simulink model "SoCesti"  (R2025a)
settings: Solver=FixedStepAuto  StartTime=0.0  StopTime=37660  FixedStep=1  RelTol=1e-3
values from neighbouring files (symbols this model uses):
  dOCV_dSOC_25 = [27.0351343549 21.2513205156 13.5820163963 10.6101110655 8.83642238875 7.64097964374 6.7848233075 6.15584045027 5.63144355991 5.17465177199 4.80430871102 4.47325692957 ... (201 elements, 1x201)]    [WSN9.mat]
  OCV_25 = [3.02032761574 3.15550328751 3.23284082089 3.29132345148 3.33894193155 3.37968767536 3.41535172799 3.44753590844 3.47691013249 3.50385034404 3.52865665021 3.55189343115 ... (201 elements, 1x201)]    [WSN9.mat]
  SOC = [0 0.005 0.01 0.015 0.02 0.025 0.03 0.035 0.04 0.045 0.05 0.055 ... (201 elements, 1x201)]    [WSN9.mat]
libraries: matrix_library x6
settings Model: Creator=lty32  LastModifiedBy=lty32
settings OptimizationCC: DefaultParameterBehavior=Inlined  EnhancedBackFolding=on  PassReuseOutputArgsThreshold=0.0  OptimizeBlockOrder=speed  DifferentSizesBufferReuse=on  OptimizationCustomize=off
settings DebuggingCC: ParameterTunabilityLossMsg=error  SFUnexpectedBacktrackingDiag=warning  SFNoUnconditionalDefaultTransitionDiag=warning
settings SFSimCC: MATLABDynamicMemAlloc=off
settings RTWCC: GenerateReport=on  BuildConfiguration=Debug  LaunchReport=on
settings CodeAppCC: ForceParamTrailComments=on  OperatorAnnotations=on  EnableCustomComments=on

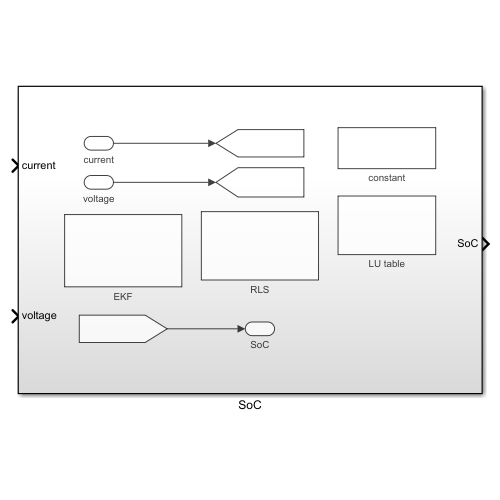
[thumbnail: Simulink's stored preview of the top-level diagram]
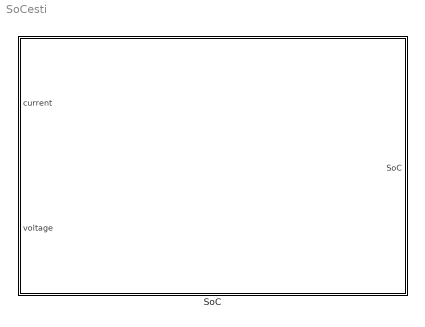
== system SoCesti ==
  SoC : Subsystem

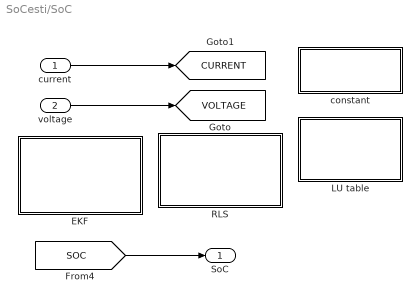
== system SoCesti/SoC ==
  current : Inport
  voltage : Inport  Port=2
  EKF : Subsystem
  LU table : Subsystem
  RLS : Subsystem
  constant : Subsystem
  SoC : Outport
  tag scope: CURRENT=global, VOLTAGE=global
  wires:
  current/1 -> [CURRENT]
  voltage/1 -> [VOLTAGE]
  [SOC] -> SoC/1

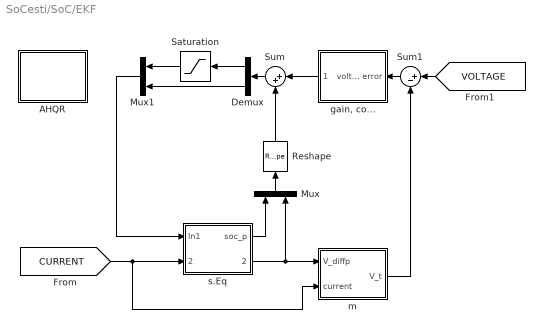
== system SoCesti/SoC/EKF ==
  AHQR : Subsystem
  Demux : Demux  Outputs=2
  Mux : Mux  Inputs=2
  Mux1 : Mux  Inputs=2
  Reshape : Reshape  OutputDimensionality=Column vector (2-D)
  Saturation : Saturate  UpperLimit=1  LowerLimit=0
  Sum : Sum  Inputs=|++
  Sum1 : Sum  Inputs=|+-
  "gain, co..." : Subsystem
  m : Subsystem
  s.Eq : Subsystem
  wires:
  [CURRENT] -> m/2(current), s.Eq/2(current)
  s.Eq/2(V_diffp) -> m/1(V_diffp), Mux/2
  Mux/1 -> Reshape/1
  Reshape/1 -> Sum/2
  Saturation/1 -> Mux1/1
  Demux/1 -> Saturation/1
  Demux/2 -> Mux1/2
  Sum/1 -> Demux/1
  Mux1/1 -> s.Eq/1(In1)
  "gain, co..."/1(1) -> Sum/1
  Sum1/1 -> "gain, co..."/1(voltage error)
  [VOLTAGE] -> Sum1/1
  s.Eq/1(soc_p) -> Mux/1
  m/1(V_t) -> Sum1/2

== system SoCesti/SoC/LU table ==
  1-D Lookup Table1 : Lookup_n-D  NumberOfTableDimensions=1  BreakpointsForDimension1=SOC  Table=OCV_25  InternalRulePriority=Speed  RndMeth=Simplest
  1-D Lookup Table4 : Lookup_n-D  NumberOfTableDimensions=1  BreakpointsForDimension1=SOC  Table=dOCV_dSOC_25  InternalRulePriority=Speed  RndMeth=Simplest
  tag scope: OCV=global, dOCV=global
  wires:
  [SOC] -> 1-D Lookup Table4/1, 1-D Lookup Table1/1
  1-D Lookup Table1/1 -> [OCV]
  1-D Lookup Table4/1 -> [dOCV]

== system SoCesti/SoC/RLS ==
  Subsystem : Subsystem
  tag scope: C1=global, R0=global, R1=global
  wires:
  Subsystem/1(r0) -> [R0]
  Subsystem/2(r1) -> [R1]
  Subsystem/3(c1) -> [C1]
  [VOLTAGE] -> Subsystem/2(voltage)
  [CURRENT] -> Subsystem/1(current)

== system SoCesti/SoC/constant ==
  "[C]" : Constant  Value=5.1344*3600  VectorParams1D=off
  sampling time [s] : Constant  VectorParams1D=off
  tag scope: dt=global, q=global
  wires:
  sampling time [s]/1 -> [dt]
  "[C]"/1 -> [q]

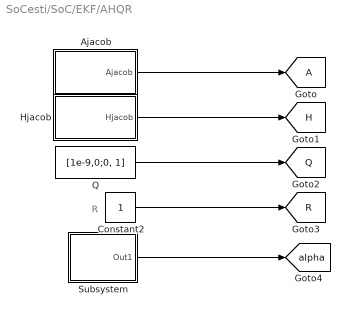
== system SoCesti/SoC/EKF/AHQR ==
  note: R
  Ajacob : Subsystem
  Constant2 : Constant  VectorParams1D=off
  Goto : Goto  TagVisibility=global
  Hjacob : Subsystem
  Q : Constant  Value=[1e-9,0;0, 1]  VectorParams1D=off
  Subsystem : Subsystem
  tag scope: H=global, Q=global, R=global, alpha=global
  wires:
  Hjacob/1(Hjacob) -> [H]
  Ajacob/1(Ajacob) -> Goto/1
  Q/1 -> [Q]
  Constant2/1 -> [R]
  Subsystem/1(Out1) -> [alpha]

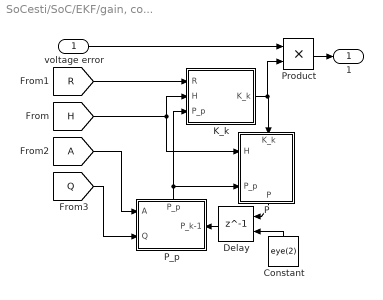
== system SoCesti/SoC/EKF/gain, co... ==
  voltage error : Inport
  Constant : Constant  Value=eye(2)  VectorParams1D=off
  Delay : Delay  DelayLength=1  InitialConditionSource=Input port  InitialCondition=0
      settings: InputPortMap=u0,p4
  From2 : From  TagVisibility=global
  K_k : Subsystem
  P : Subsystem
      settings: PortSchema="{\"entries\":[{\"content\":{\"sides\":[{\"content\":{\"connectorIds\":[\"In1\"]},\"type\":\"ConnectorPlacement.EquallySpacedRectSide\",\"uuid\":\"6f300193-b535-4daf-8653-539d9fbd6dc4\"},{\"content\":{\"connectorIds\":[\"Out1\"],\"side\":\"RIGHT\"},\"type\":\"ConnectorPlacement.EquallySpacedRectSide\",\"uuid\":\"87a1046a-ef69-4257-b5a0-a19886caf6fd\"},{\"content\":{\"connectorIds\":[\"In2\",\"In3\"],\"side\":\"TOP\"},\"type\":\"ConnectorPlacement.EquallySpacedRectSide\",\"uuid\":\"b6a053fa-a3d4-4df4-83df-54ae82e90296\"},{\"content\":{\"side\":\"BOTTOM\"},\"type\":\"ConnectorPlacement.EquallySpacedRectSide\",\"uuid\":\"c9b75463-d757-4499-9316-63b6258cebf3\"}]},\"type\":\"ConnectorPlacement.EquallySpacedConnector\",\"uuid\":\"417e791e-5d64-4019-ac72-5f0d428a58a7\"}],\"packageUris\":[\"http://schema.mathworks.com/mf0/Connector/R2020b\"],\"version\":\"1.0\"}"
  P_p : Subsystem
      settings: PortSchema="{\"entries\":[{\"content\":{\"sides\":[{\"content\":{\"connectorIds\":[\"In1\"]},\"type\":\"ConnectorPlacement.EquallySpacedRectSide\",\"uuid\":\"6f300193-b535-4daf-8653-539d9fbd6dc4\"},{\"content\":{\"connectorIds\":[\"In2\",\"In3\"],\"side\":\"RIGHT\"},\"type\":\"ConnectorPlacement.EquallySpacedRectSide\",\"uuid\":\"87a1046a-ef69-4257-b5a0-a19886caf6fd\"},{\"content\":{\"connectorIds\":[\"Out1\"],\"side\":\"TOP\"},\"type\":\"ConnectorPlacement.EquallySpacedRectSide\",\"uuid\":\"b6a053fa-a3d4-4df4-83df-54ae82e90296\"}]},\"type\":\"ConnectorPlacement.EquallySpacedConnector\",\"uuid\":\"417e791e-5d64-4019-ac72-5f0d428a58a7\"}],\"packageUris\":[\"http://schema.mathworks.com/mf0/Connector/R2020b\"],\"version\":\"1.0\"}"
  Product : Product
  1 : Outport
  wires:
  P/1(P) -> Delay/1
  K_k/1(K_k) -> P/1(K_k), Product/2
  P_p/1(P_p) -> K_k/3(P_p), P/3(P_p)
  [R] -> K_k/1(R)
  [H] -> K_k/2(H), P/2(H)
  [Q] -> P_p/3(Q)
  voltage error/1 -> Product/1
  From2/1 -> P_p/2(A)
  Delay/1 -> P_p/1(P_k-1)
  Constant/1 -> Delay/2
  Product/1 -> 1/1

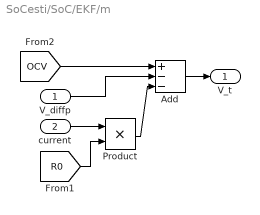
== system SoCesti/SoC/EKF/m ==
  V_diffp : Inport
  current : Inport  Port=2
  Add : Sum  Inputs=+--
  Product : Product
  V_t : Outport
  wires:
  Add/1 -> V_t/1
  [OCV] -> Add/1
  V_diffp/1 -> Add/2
  [R0] -> Product/2
  current/1 -> Product/1
  Product/1 -> Add/3

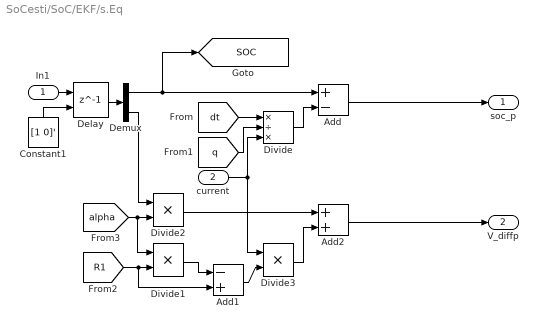
== system SoCesti/SoC/EKF/s.Eq ==
  In1 : Inport
  current : Inport  Port=2
  Add : Sum  Inputs=+-
  Add1 : Sum  Inputs=-+
  Add2 : Sum
  Constant1 : Constant  Value=[1 0]'  VectorParams1D=off
  Delay : Delay  DelayLength=1  InitialConditionSource=Input port  InitialCondition=0
      settings: InputPortMap=u0,p4
  Demux : Demux  Outputs=2
  Divide : Product  Inputs=*/*
  Divide1 : Product  Inputs=**
  Divide2 : Product  Inputs=**
  Divide3 : Product  Inputs=**
  soc_p : Outport
  V_diffp : Outport  Port=2
  tag scope: SOC=global
  wires:
  current/1 -> Divide3/1, Divide/3
  [dt] -> Divide/1
  [q] -> Divide/2
  Divide/1 -> Add/2
  Demux/1 -> [SOC], Add/1
  Add/1 -> soc_p/1
  Add2/1 -> V_diffp/1
  In1/1 -> Delay/1
  Delay/1 -> Demux/1
  Constant1/1 -> Delay/2
  [R1] -> Add1/2, Divide1/2
  [alpha] -> Divide1/1, Divide2/2
  Demux/2 -> Divide2/1
  Divide1/1 -> Add1/1
  Divide2/1 -> Add2/1
  Add1/1 -> Divide3/2
  Divide3/1 -> Add2/2

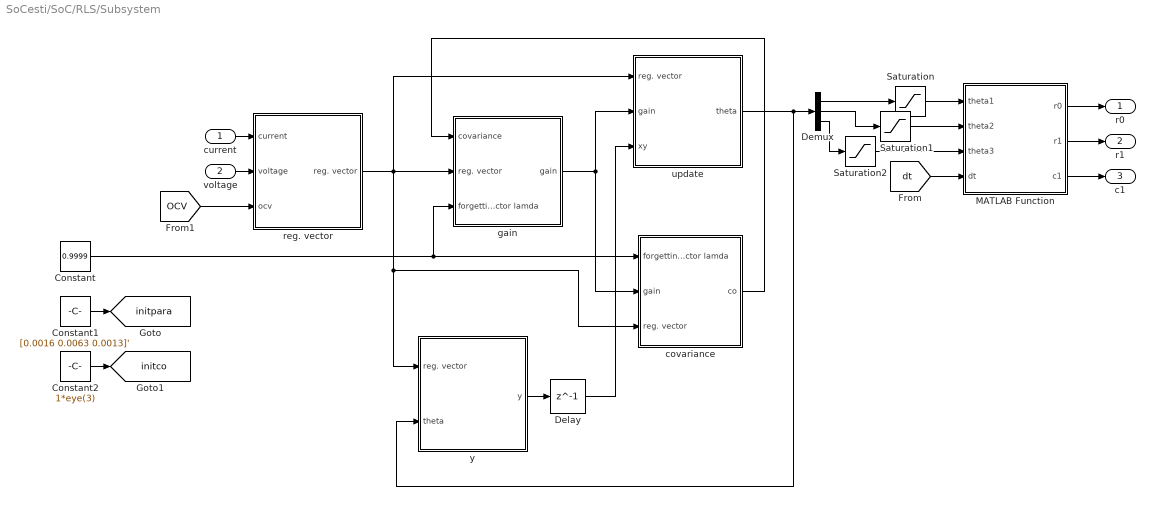
== system SoCesti/SoC/RLS/Subsystem ==
  current : Inport
  voltage : Inport  Port=2
  Constant : Constant  Value=0.9999
  Constant1 : Constant  Value=[0.0016 0.0063 0.0013]'  VectorParams1D=off
  Constant2 : Constant  Value=1*eye(3)  VectorParams1D=off
  Delay : Delay  DelayLength=1  InitialCondition=0
  Demux : Demux  Outputs=3
  MATLAB Function : MATLAB Function  TreatAsAtomicUnit=on
  Saturation : Saturate  UpperLimit=0.1  LowerLimit=0.000001  LinearizeAsGain=off
  Saturation1 : Saturate  LowerLimit=0.000001
  Saturation2 : Saturate  LowerLimit=0.000001
  covariance : Subsystem
  gain : Subsystem
  reg. vector : Subsystem
  update : Subsystem
  y : Subsystem
  r0 : Outport
  r1 : Outport  Port=2
  c1 : Outport  Port=3
  tag scope: initco=global, initpara=global
  wires:
  current/1 -> reg. vector/1(current)
  voltage/1 -> reg. vector/2(voltage)
  MATLAB Function/1(r0) -> r0/1
  MATLAB Function/2(r1) -> r1/1
  MATLAB Function/3(c1) -> c1/1
  [dt] -> MATLAB Function/4(dt)
  update/1(theta) -> y/2(theta), Demux/1
  reg. vector/1(reg. vector) -> y/1(reg. vector), covariance/3(reg. vector), update/1(reg. vector), gain/2(reg. vector)
  covariance/1(co) -> gain/1(covariance)
  gain/1(gain) -> covariance/2(gain), update/2(gain)
  Constant/1 -> gain/3(forgetting factor lamda), covariance/1(forgetting factor lamda)
  Constant1/1 -> [initpara]
  Constant2/1 -> [initco]
  [OCV] -> reg. vector/3(ocv)
  Demux/1 -> Saturation/1
  Saturation/1 -> MATLAB Function/1(theta1)
  Saturation1/1 -> MATLAB Function/2(theta2)
  Demux/2 -> Saturation1/1
  Saturation2/1 -> MATLAB Function/3(theta3)
  Demux/3 -> Saturation2/1
  y/1(y) -> Delay/1
  Delay/1 -> update/3(xy)

== system SoCesti/SoC/EKF/AHQR/Ajacob ==
  Add : Sum
  Constant : Constant  Value=[0, 0; 0, 1]
  Constant1 : Constant  Value=[1, 0; 0, 0]
  Product : Product
  Ajacob : Outport
  wires:
  Add/1 -> Ajacob/1
  Product/1 -> Add/1
  Constant1/1 -> Add/2
  [alpha] -> Product/2
  Constant/1 -> Product/1

== system SoCesti/SoC/EKF/AHQR/Hjacob ==
  Add : Sum  Inputs=+-
  Constant : Constant  Value=[1 0]  VectorParams1D=off
  Constant1 : Constant  Value=[0 1]  VectorParams1D=off
  Product : Product
  Hjacob : Outport
  wires:
  Add/1 -> Hjacob/1
  Product/1 -> Add/1
  Constant1/1 -> Add/2
  [dOCV] -> Product/2
  Constant/1 -> Product/1

== system SoCesti/SoC/EKF/AHQR/Subsystem ==
  Constant : Constant  Value=-1  VectorParams1D=off
  Divide : Product  Inputs=**//
  Math Function : Math  OutputSignalType=real
  Out1 : Outport
  wires:
  [C1] -> Divide/4
  [R1] -> Divide/3
  [dt] -> Divide/2
  Constant/1 -> Divide/1
  Divide/1 -> Math Function/1
  Math Function/1 -> Out1/1

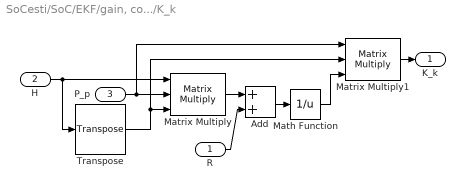
== system SoCesti/SoC/EKF/gain, co.../K_k ==
  R : Inport
  H : Inport  Port=2
  P_p : Inport  Port=3
  Add : Sum
  Math Function : Math  Operator=reciprocal
  Matrix Multiply : Product  Inputs=3  Multiplication=Matrix(*)
  Matrix Multiply1 : Product  Inputs=3  Multiplication=Matrix(*)
  Transpose : matrix_library/Transpose
  K_k : Outport
  wires:
  P_p/1 -> Matrix Multiply1/1, Matrix Multiply/2
  H/1 -> Transpose/1, Matrix Multiply/1
  Transpose/1 -> Matrix Multiply/3, Matrix Multiply1/2
  Matrix Multiply/1 -> Add/1
  R/1 -> Add/2
  Matrix Multiply1/1 -> K_k/1
  Add/1 -> Math Function/1
  Math Function/1 -> Matrix Multiply1/3

== system SoCesti/SoC/EKF/gain, co.../P ==
  K_k : Inport
  H : Inport  Port=2
  P_p : Inport  Port=3
  Matrix Multiply : Product  Inputs=3  Multiplication=Matrix(*)
  Subtract : Sum  Inputs=+-
  P : Outport
  wires:
  K_k/1 -> Matrix Multiply/1
  H/1 -> Matrix Multiply/2
  P_p/1 -> Subtract/1, Matrix Multiply/3
  Matrix Multiply/1 -> Subtract/2
  Subtract/1 -> P/1

== system SoCesti/SoC/EKF/gain, co.../P_p ==
  P_k-1 : Inport
  A : Inport  Port=2
  Q : Inport  Port=3
  Add : Sum
  Matrix Multiply : Product  Inputs=3  Multiplication=Matrix(*)
  Transpose : matrix_library/Transpose
  P_p : Outport
  wires:
  P_k-1/1 -> Matrix Multiply/2
  Q/1 -> Add/2
  A/1 -> Transpose/1, Matrix Multiply/1
  Matrix Multiply/1 -> Add/1
  Transpose/1 -> Matrix Multiply/3
  Add/1 -> P_p/1

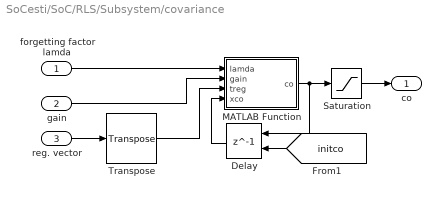
== system SoCesti/SoC/RLS/Subsystem/covariance ==
  forgetting factor lamda : Inport
  gain : Inport  Port=2
  reg. vector : Inport  Port=3
  Delay : Delay  DelayLength=1  InitialConditionSource=Input port  InitialCondition=0
      settings: InputPortMap=u0,p4
  MATLAB Function : MATLAB Function  TreatAsAtomicUnit=on
  Saturation : Saturate  UpperLimit=inf  LowerLimit=0.000001  LinearizeAsGain=off
  Transpose : matrix_library/Transpose
  co : Outport
  wires:
  forgetting factor lamda/1 -> MATLAB Function/1(lamda)
  gain/1 -> MATLAB Function/2(gain)
  reg. vector/1 -> Transpose/1
  Transpose/1 -> MATLAB Function/3(treg)
  MATLAB Function/1(co) -> Saturation/1, Delay/1
  Delay/1 -> MATLAB Function/4(xco)
  [initco] -> Delay/2
  Saturation/1 -> co/1

== system SoCesti/SoC/RLS/Subsystem/gain ==
  covariance : Inport
  reg. vector : Inport  Port=2
  forgetting factor lamda : Inport  Port=3
  Delay : Delay  DelayLength=1  InitialCondition=0
  MATLAB Function : MATLAB Function  TreatAsAtomicUnit=on
  Transpose : matrix_library/Transpose
  gain : Outport
  wires:
  forgetting factor lamda/1 -> MATLAB Function/1(lamda)
  reg. vector/1 -> MATLAB Function/2(reg), Transpose/1
  Transpose/1 -> MATLAB Function/3(treg)
  covariance/1 -> Delay/1
  Delay/1 -> MATLAB Function/4(xco)
  MATLAB Function/1(gain) -> gain/1

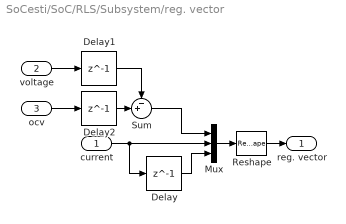
== system SoCesti/SoC/RLS/Subsystem/reg. vector ==
  current : Inport
  voltage : Inport  Port=2
  ocv : Inport  Port=3
  Delay : Delay  DelayLength=1  InitialCondition=0
  Delay1 : Delay  DelayLength=1  InitialCondition=0
  Delay2 : Delay  DelayLength=1  InitialCondition=0
  Mux : Mux  Inputs=3
  Reshape : Reshape  OutputDimensionality=Column vector (2-D)
  Sum : Sum  Inputs=-+|
  reg. vector : Outport
  wires:
  Mux/1 -> Reshape/1
  Reshape/1 -> reg. vector/1
  current/1 -> Delay/1, Mux/2
  voltage/1 -> Delay1/1
  Delay1/1 -> Sum/1
  ocv/1 -> Delay2/1
  Delay2/1 -> Sum/2
  Delay/1 -> Mux/3
  Sum/1 -> Mux/1

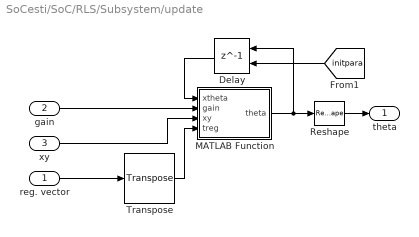
== system SoCesti/SoC/RLS/Subsystem/update ==
  reg. vector : Inport
  gain : Inport  Port=2
  xy : Inport  Port=3
  Delay : Delay  DelayLength=1  InitialConditionSource=Input port  InitialCondition=0
      settings: InputPortMap=u0,p4
  MATLAB Function : MATLAB Function  TreatAsAtomicUnit=on
  Reshape : Reshape  OutputDimensionality=Column vector (2-D)
  Transpose : matrix_library/Transpose
  theta : Outport
  wires:
  gain/1 -> MATLAB Function/2(gain)
  xy/1 -> MATLAB Function/3(xy)
  reg. vector/1 -> Transpose/1
  Transpose/1 -> MATLAB Function/4(treg)
  MATLAB Function/1(theta) -> Reshape/1, Delay/1
  [initpara] -> Delay/2
  Reshape/1 -> theta/1
  Delay/1 -> MATLAB Function/1(xtheta)

== system SoCesti/SoC/RLS/Subsystem/y ==
  reg. vector : Inport
  theta : Inport  Port=2
  Matrix Multiply : Product  Multiplication=Matrix(*)
  Transpose : matrix_library/Transpose
  y : Outport
  wires:
  reg. vector/1 -> Transpose/1
  Transpose/1 -> Matrix Multiply/1
  theta/1 -> Matrix Multiply/2
  Matrix Multiply/1 -> y/1

== matlab function SoCesti/SoC/RLS/Subsystem/MATLAB Function ==
  data: theta1 input; theta2 input; theta3 input; r0 output; r1 output; c1 output; dt input
function [r0, r1, c1]= fcn(theta1, theta2, theta3, dt)

r0 = theta2;
r1 = (theta3 + (theta1*theta2))/(1 - theta1);
c1 = -(dt*(1 - theta1))/((theta3 + (theta1*theta2))*log(theta1));

== matlab function SoCesti/SoC/RLS/Subsystem/covariance/MATLAB Function ==
  data: lamda input; co output; gain input; treg input; xco input
function co = fcn(lamda, gain, treg, xco)

co = (1/lamda)*(xco - gain*treg*xco);

== matlab function SoCesti/SoC/RLS/Subsystem/gain/MATLAB Function ==
  data: lamda input; reg input; gain output; treg input; xco input
function gain = fcn(lamda, reg, treg, xco)

gain = (xco*reg)/(lamda + (treg*xco*reg));

== matlab function SoCesti/SoC/RLS/Subsystem/update/MATLAB Function ==
  data: xtheta input; theta output; gain input; xy input; treg input
function theta = fcn(xtheta, gain, xy, treg)

theta = xtheta + gain*(xy-(treg*xtheta));
